simulink model "soft22_sim"  (Simulink 7.3)
settings: Solver=ode15s  StartTime=0.0  StopTime=5  FixedStep=0.0005  MaxStep=0.001  RelTol=0.01  AbsTol=0.01
values from neighbouring files (symbols this model uses):
  init_dq1 = [0.0; 0.0]    [soft22_ini.m]
  init_dq2 = [0.0; 0.0]    [soft22_ini.m]
  init_q1 = IN(16:17)    [soft22.m]    (also in soft22_ini.m = [2.1670; -1.75160])
  init_q2 = IN(18:19)    [soft22.m]    (also in soft22_ini.m = [0.9745;  1.75160])
settings Model: Creator=tahara  LastModifiedBy=tahara  ExtModeTrigMode=oneshot  ExtModeArmWhenConnect=off
settings DataIOCC: LimitDataPoints=off  SignalLoggingName=sigsOut
settings OptimizationCC: BooleanDataType=off  InitFltsAndDblsToZero=on
settings DebuggingCC: SaveWithParameterizedLinksMsg=none  SignalResolutionControl=TryResolveAllWithWarning  SolverPrmCheckMsg=none  MultiTaskDSMMsg=warning  MultiTaskCondExecSysMsg=none  StrictBusMsg=None
settings HardwareCC: TargetUnknown=on
settings RTWCC: IncludeERTFirstTime=on
settings GRTTargetCC: TargetFcnLib=ansi_tfl_tmw.mat  ModelReferenceCompliant=off  MatFileLogging=off

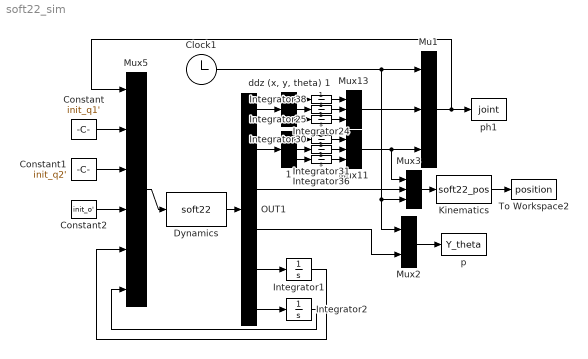
== system soft22_sim ==
  " 1" : Demux  Outputs=[2 2 3]
  Clock1 : Clock
      settings: Decimation=10
  Constant : Constant  Value=init_q1'  OutDataType=sfix(16)  OutScaling=2^0
  Constant1 : Constant  Value=init_q2'  OutDataType=sfix(16)  OutScaling=2^0
  Constant2 : Constant  Value=init_o'  OutDataType=sfix(16)  OutScaling=2^0
  Dynamics : MATLABFcn  MATLABFcn=soft22  OutputDimensions=35
  Integrator1 : Integrator
  Integrator2 : Integrator  InitialCondition=[0 0]
  Integrator24 : Integrator  InitialCondition=init_dq2'
  Integrator25 : Integrator  InitialCondition=init_do'
  Integrator30 : Integrator  InitialCondition=init_q1'
  Integrator31 : Integrator  InitialCondition=init_q2'
  Integrator36 : Integrator  InitialCondition=init_o'
  Integrator38 : Integrator  InitialCondition=init_dq1'
  Kinematics : MATLABFcn  MATLABFcn=soft22_pos  OutputDimensions=36  Output1D=off
  Mu1 : Mux  Inputs=[1 7 7]
  Mux11 : Mux  Inputs=[2 2 3]
  Mux13 : Mux  Inputs=[2 2 3]
  Mux2 : Mux  Inputs=[1 14]
  Mux3 : Mux  Inputs=[7 4 1]
  Mux5 : Mux  Inputs=[15 2 2 3 1 2]
  OUT1 : Demux  Outputs=[7 7 4 14 1 2]
  To Workspace2 : ToWorkspace  VariableName=position  SampleTime=0.033  SaveFormat=Array
  "ddz (x, y, theta) 1" : Demux  Outputs=[2 2 3]
  p : ToWorkspace  VariableName=Y_theta  SampleTime=-1  SaveFormat=Array
  ph1 : ToWorkspace  VariableName=joint  SampleTime=-1  SaveFormat=Array
  wires:
  Dynamics/1 -> OUT1/1
  "ddz (x, y, theta) 1"/1 -> Integrator38/1
  "ddz (x, y, theta) 1"/2 -> Integrator24/1
  "ddz (x, y, theta) 1"/3 -> Integrator25/1
  Integrator25/1 -> Mux13/3
  Integrator24/1 -> Mux13/2
  Integrator38/1 -> Mux13/1
  " 1"/1 -> Integrator30/1
  Integrator30/1 -> Mux11/1
  Integrator31/1 -> Mux11/2
  Integrator36/1 -> Mux11/3
  " 1"/2 -> Integrator31/1
  " 1"/3 -> Integrator36/1
  Mux2/1 -> p/1
  Clock1/1 -> Mu1/1, Mux3/3, Mux2/1
  Mu1/1 -> ph1/1, Mux5/1
  Kinematics/1 -> To Workspace2/1
  OUT1/1 -> "ddz (x, y, theta) 1"/1
  Mux13/1 -> Mu1/2
  OUT1/2 -> " 1"/1
  Mux11/1 -> Mu1/3, Mux3/1
  Mux3/1 -> Kinematics/1
  OUT1/3 -> Mux3/2
  OUT1/4 -> Mux2/2
  Mux5/1 -> Dynamics/1
  Constant/1 -> Mux5/2
  Constant1/1 -> Mux5/3
  Constant2/1 -> Mux5/4
  Integrator1/1 -> Mux5/5
  Integrator2/1 -> Mux5/6
  OUT1/5 -> Integrator1/1
  OUT1/6 -> Integrator2/1
